simulink model "practica2_sim"  (R2022b)
settings: Solver=VariableStepAuto  StartTime=0.0  StopTime=20.0  RelTol=1e-3
values from neighbouring files (symbols this model uses):
  b1 = 500    [practica2.m]
  b2 = 500    [practica2.m]
  k = 100    [practica2.m]
  m1 = 1000    [practica2.m]
  m2 = 3000    [practica2.m]
settings Model: Creator=Fran  LastModifiedBy=Fran

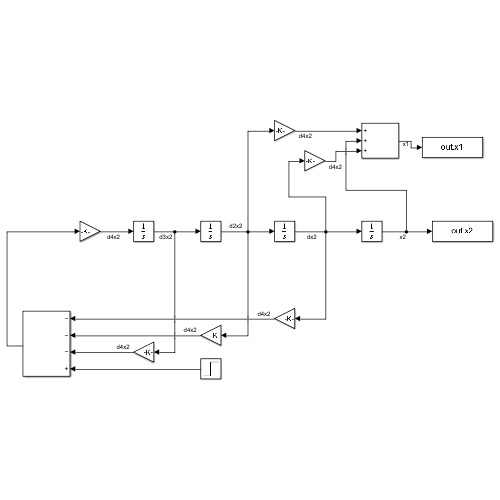
[thumbnail: Simulink's stored preview of the top-level diagram]
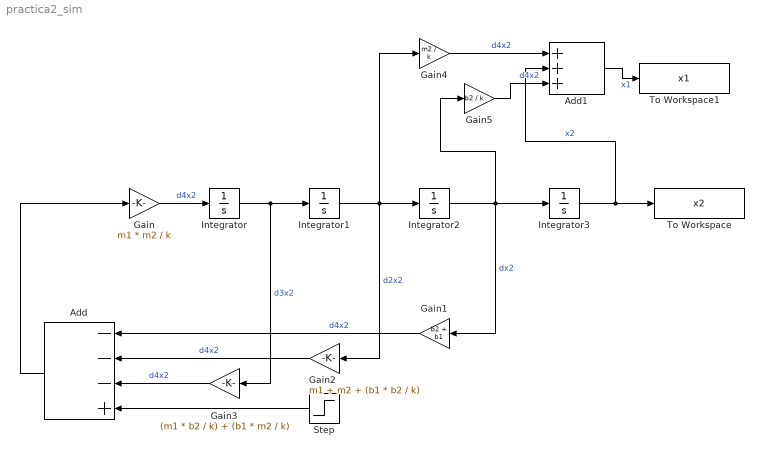
== system practica2_sim ==
  Add : Sum  Inputs=---+
  Add1 : Sum  Inputs=+++
  Gain : Gain  Gain=m1 * m2 / k
  Gain1 : Gain  Gain=b2 + b1
  Gain2 : Gain  Gain=m1 + m2 + (b1 * b2 / k)
  Gain3 : Gain  Gain=(m1 * b2 / k) + (b1 * m2 / k)
  Gain4 : Gain  Gain=m2 / k
  Gain5 : Gain  Gain=b2 / k
  Integrator{,1..3} (4 alike) : Integrator
  Step : Step  Time=0.1  After=500  SampleTime=0
  To Workspace : ToWorkspace  VariableName=x2  SampleTime=-1
  To Workspace1 : ToWorkspace  VariableName=x1  SampleTime=-1
  wires:
  Integrator/1 -> Gain3/1, Integrator1/1  "d3x2"
  Integrator1/1 -> Gain4/1, Gain2/1, Integrator2/1  "d2x2"
  Integrator2/1 -> Gain5/1, Gain1/1, Integrator3/1  "dx2"
  Integrator3/1 -> Add1/2, To Workspace/1  "x2"
  Gain/1 -> Integrator/1  "d4x2"
  Add/1 -> Gain/1
  Gain1/1 -> Add/1  "d4x2"
  Gain2/1 -> Add/2  "d4x2"
  Gain3/1 -> Add/3  "d4x2"
  Step/1 -> Add/4
  Add1/1 -> To Workspace1/1  "x1"
  Gain4/1 -> Add1/1  "d4x2"
  Gain5/1 -> Add1/3  "d4x2"
